simulink model "overalldesign_change_down"  (R2025b)
settings: Solver=ode4  StartTime=0.0  StopTime=1200  FixedStep=0.01  MaxStep=0.01  RelTol=1e-4
PreLoadFcn:
  | % Component data matrix: [present, weight_kg, MX_kgmm, MY_kgmm, MZ_kgmm]
  | % Rows 1-28 correspond to Excel rows 2-29
  | comp_data_mat = [
  |   1, 80,     147543.64,  -0.88,    -1622.36;    % 底盘
  |   1, 60,      73274.04, -169.26,    3359.46;    % 轮胎
  |   0,  0,             0,       0,         0;    % 前后桥(不在位)
  |   1, 45,      99639.05,  -0.495,   35241.39;    % 蒙皮
  |   1, 159,    308512.15, -0.0298,   72044.97;    % 结构骨架
  |   1, 93,     214584.20,  -1.023,   85225.94;    % 折叠机构
  |   1, 113.92, 269830.46, -1.2531,  107552.44;    % 支臂
  |   1, 45,       1371.65, -531.27,   17662.14;    % 内饰
  |   1, 13.86,   34638.76, -0.1525,   13254.18;    % 电机底座
  |   1, 30,      69816.09,   -0.33,   26989.32;    % 飞行体
  |   1, 316,    803427.47,       0,   33092.78;    % 动力电池1
  |   0, 316,            0,       0,         0;    % 动力电池2(不在位)
  |   1, 30,      75059.94,    0.21,   37410.81;    % 旋翼
  |   1, 141,    353019.16,  -1.551,  161459.10;    % 电机
  |   1, 33,      82253.26,   -0.33,   27077.13;    % 电调
  |   1, 15,             0,       0,         0;    % PDU
  |   0, 10,             0,       0,         0;    % 导线(不在位)
  |   0,  0,             0,       0,         0;    % (空)
  |   0, 90,             0,       0,         0;    % 左商载(不在位)
  |   0, 90,             0,       0,         0;    % 右商载(不在位)
  |   0, 32,             0,       0,         0;    % 飞控运控(不在位)
  | 
  | ];
  | % Lift center [X; Y; Z] in mm
  | lift_center_vec = [2506.477; 0; 1258.273];
  | % Route parameters are set directly in top-level Constant blocks:
  | %   route_mode, takeoff, hover, line_cruise, circle_cruise, land
model workspace (MAT data in the model file):
  CS_duct_lift_slew_rate = 7031250
  CS_main_rotor_slew_rate = 1567.1641791
  CS_max_acc_xy = 5
  CS_max_acc_z_down = 5
  CS_max_acc_z_up = 5
  CS_max_jerk_xy = 20
  CS_max_jerk_z_down = 20
  CS_max_jerk_z_up = 20
  CS_max_vel_xy = 20
  CS_max_vel_z_down = 20
  CS_max_vel_z_up = 20
  CS_motor_tau_duct = 0.07
  CS_motor_tau_main = 0.336
  Kd_rate_rp = 12
  Kd_rate_y = 8
  Kd_vel_xy = 1.5
  Kd_vel_z = 1
  Ki_rate_rp = 4
  Ki_rate_y = 10
  Ki_vel_xy = 0.02
  Ki_vel_z = 0.05
  Kp_att_rp = 2.5
  Kp_att_tilt = 2.5
  Kp_att_y = 1.5
  Kp_att_yaw = 1.5
  Kp_pos_xy = 0.4
  Kp_pos_z = 1
  Kp_rate_rp = 300
  Kp_rate_y = 200
  Kp_vel_xy = 1.5
  Kp_vel_z = 1.5
  P.source.audit_file = 'main_model_param_audit.xlsx'
  P.source.note = 'CG and motor positions are default snapshots here. The pipeline updates them from Excel before simulation.'
  P.model.stop_time_s = 60
  P.model.cg_calculation_commented = 'on'
  P.route.mode = 2
  P.fault.id = 0
  P.mass_kg = 1200
  P.inertia_kgm2 = [3959.6  0  0; 0  3041.4  0; 0  0  2640.2]
  P.cg_offset_m = [0.038293; -0.0063; 0.28227]
  P.environment.gravity_mps2 = 9.81
  P.environment.rho_kgpm3 = 1.225
  P.environment.g = 9.81
  P.environment.rho = 1.225
  P.battery.total_Wh = 80000
  P.battery.usable_ratio = 0.8
  P.motor.efficiency = 0.85
  P.rotor.count = 6
  P.rotor.radius_m = 1.3
  P.rotor.blade_num = 2
  P.rotor.chord_avg_m = 0.18
  P.rotor.pos_m = [2.624  -2.228  -0.465; 2.624  2.228  -0.465; 0  -2.235  0; 0  2.235  0; -2.599  -2.231  -0.464; -2.599  2.231  -0.464]
  P.rotor.spin_dir = [1; -1; -1; 1; 1; -1]
  P.rotor.kF_N_per_radps2 = 0.00141483
  P.rotor.kM_Nm_per_radps2 = 0.000167666
  P.rotor.power_coeff_W_per_radps3 = 1.74522e-05
  P.rotor.kF = 0.00141483
  P.rotor.kM = 0.000167666
  P.rotor.speed_max_radps = 1770
  P.rotor.speed_margin_radps = 1600
  P.duct.power_coeff_W_per_radps3 = 5.12708e-07
  P.duct.kF_N_per_radps2 = 4.54e-05
  P.duct.kF = 4.54e-05
  P.duct.pos_m = [3  0  0; 3  0  0]
  P.duct.force_dir = [0  -1  0; 0  1  0]
  P.mixer.T_hover_N = 11772
  P.mixer.W_hover_radps = 1177.6
  P.mixer.ref_col_norms = [2.014; 2.149; 2.4849; 2.4849]
  P.control.max_tilt_deg = 20
  P.control.max_tilt_rad = 0.349065850399
  P.review.current_6DoF_mass_kg = 1208.5
  P.review.current_Perf_Calc_mass_kg = 1208.5
  P.review.GravBlock_mass_kg = 1200
  P.review.Accel2Attitude_mass_kg = 1200
  P.review.model_workspace_cg_offset_m = [0.25; 0; 0.62]
  P.review.model_workspace_motor_pos_m = [2.592  -2.306  0; 2.592  2.306  0; 0  -2.505  0; 0  2.505  0; -2.592  -2.306  0; -2.592  2.306  0]
  T_hover = 11772
  V_descent = []
  W_hover = 1194
  W_margin = 1600
  cg_offset_m = [0.038293; -0.0063; 0.28227]
  cg_x_delta_m = 0
  climbRate_mps = 5
  cruiseSpeed_mps = 20
  descentRate_mps = 5
  duct_dir = [0  -1  0; 0  1  0]
  duct_pos_0 = [3  0  0; 3  0  0]
  fault_id = 0
  fault_mask = [0; 0; 0; 0; 0; 0; 0; 0]
  hover_x = 0
  hover_y = 0
  hover_yaw = 0
  hover_z = -120
  inertia_kgm2 = [3959.6  0  0; 0  3041.4  0; 0  0  2640.2]
  kF = 0.0013767
  kF_duct = 4.54e-05
  kM = 0.000164967
  kM_coeff = 1.72621225e-05
  kM_duct = 4.896e-06
  kM_duct_coeff = 5.12708e-07
  k_yaw_weight = 0.5
  mass_kg = 1200
  motor_coord = [2.624  -2.228  -0.465; 2.624  2.228  -0.465; 0  -2.235  0; 0  2.235  0; -2.599  -2.231  -0.464; -2.599  2.231  -0.464; 3  0  0; 3  0  0]
  motor_dir = [1; -1; -1; 1; 1; -1]
  motor_efficiency = 0.9016
  motor_pos_0 = [2.624  -2.228  -0.465; 2.624  2.228  -0.465; 0  -2.235  0; 0  2.235  0; -2.599  -2.231  -0.464; -2.599  2.231  -0.464]
  offline_opt_applyBestToModel = 1
  offline_opt_maxEvaluations = 10
  offline_opt_method = 'auto'
  offline_opt_saveBestToModel = 0
  offline_opt_updateDiagramAfterBest = 1
  perf_battery_Wh = 80000
  perf_blade_num = 2
  perf_chord_avg = 0.18
  perf_mass_kg = 1200
  perf_rho = 1.225
  perf_rotor_num = 6
  perf_rotor_radius = 1.3
  perf_usable_ratio = 0.8
  speed_max_radps = 1750
  tau_limit_rp = 2000
  tau_limit_y = 1000
  thrust_degrade = 0.7
libraries: slpidlib x6, aerolibprivatev1p5 x1, dspnetwork x1
(part 1 of 2)
settings Model: Creator=admin  LastModifiedBy=91390
settings SolverCC: ZeroCrossControl=DisableAll

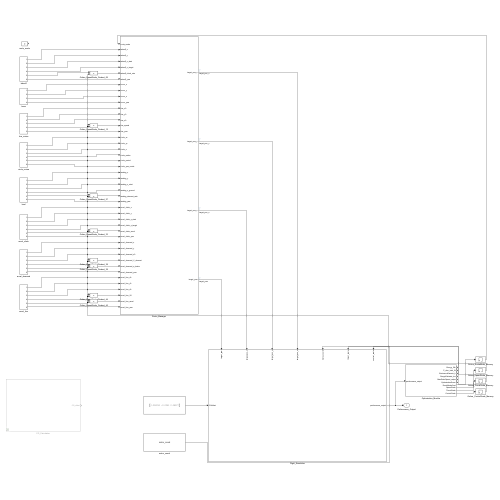
[thumbnail: Simulink's stored preview of the top-level diagram]
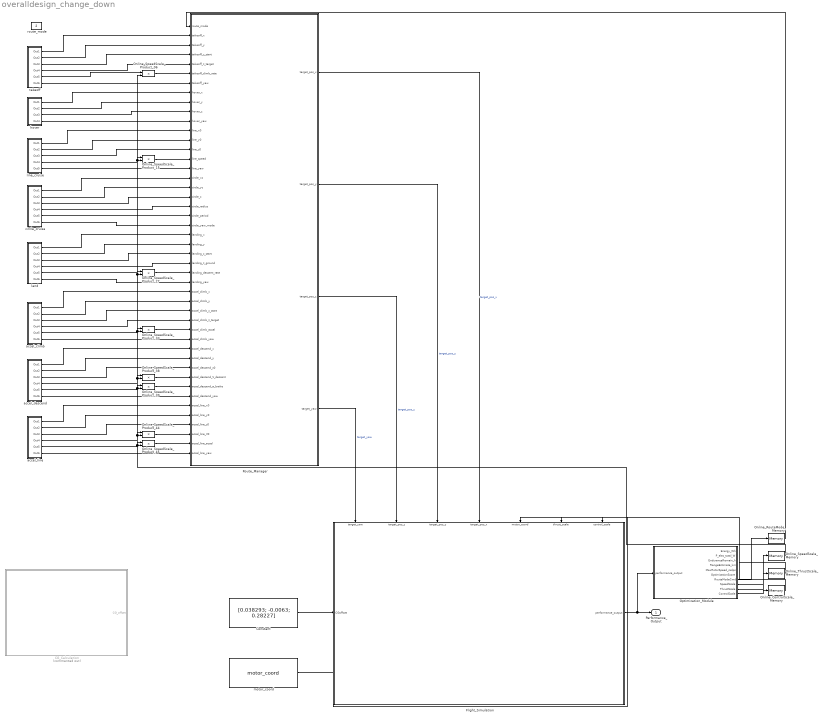
== system overalldesign_change_down ==
  CG_Calculation : Subsystem  Commented=on
  Constant : Constant  Value=[0.038293; -0.0063; 0.28227]
  Flight_Simulation : Subsystem
      settings: PortSchema="{\"entries\":[{\"content\":{\"sides\":[{\"content\":{\"connectorIds\":[\"In1\"]},\"type\":\"ConnectorPlacement.EquallySpacedRectSide\",\"uuid\":\"5deb5f2c-62ad-40f5-b613-353336255dba\"},{\"content\":{\"connectorIds\":[\"Out1\"],\"side\":\"RIGHT\"},\"type\":\"ConnectorPlacement.EquallySpacedRectSide\",\"uuid\":\"a56ec260-326c-4a45-a418-c08f727a598e\"},{\"content\":{\"connectorIds\":[\"In2\",\"In3\",\"In4\",\"In5\",\"In6\",\"In7\",\"In8\"],\"side\":\"TOP\"},\"type\":\"ConnectorPlacement.EquallySpacedRectSide\",\"uuid\":\"b9e0438d-138c-455b-afb0-6983736d76da\"}]},\"type\":\"ConnectorPlacement.EquallySpacedConnector\",\"uuid\":\"d5d418e6-8e97-46b2-8c41-4077eef2ab5a\"}],\"packageUris\":[\"http://schema.mathworks.com/mf0/Connector/R2020b\"],\"version\":\"1.0\"}"
  Online_ControlScale_Memory : Memory  InitialCondition=1
  Online_RouteMode_Memory : Memory  InitialCondition=1
  Online_SpeedScale_Memory : Memory  InitialCondition=1
  Online_SpeedScale_Product_06 : Product
  Online_SpeedScale_Product_{15,27,33,38..39,44..45} (7 alike) : Product
  Online_ThrustScale_Memory : Memory  InitialCondition=1
  Optimization_Module : Subsystem
  Route_Manager : Subsystem
  accel_climb : Subsystem
  accel_descend : Subsystem
  accel_line : Subsystem
  circle_cruise : Subsystem
  hover : Subsystem
  land : Subsystem
  line_cruise : Subsystem
  motor_coord : Constant  Value=motor_coord
  route_mode : Constant  Value=2
  takeoff : Subsystem
  Performance_Output : Outport
  wires:
  line_cruise/5(Out5) -> Route_Manager/16(line_yaw)
  takeoff/4(Out4) -> Route_Manager/5(takeoff_z_target)
  takeoff/1(Out1) -> Route_Manager/2(takeoff_x)
  circle_cruise/2(Out2) -> Route_Manager/18(circle_yc)
  takeoff/6(Out6) -> Route_Manager/7(takeoff_yaw)
  takeoff/2(Out2) -> Route_Manager/3(takeoff_y)
  accel_line/6(Out6) -> Route_Manager/46(accel_line_yaw)
  takeoff/3(Out3) -> Route_Manager/4(takeoff_z_start)
  hover/1(Out1) -> Route_Manager/8(hover_x)
  hover/2(Out2) -> Route_Manager/9(hover_y)
  hover/3(Out3) -> Route_Manager/10(hover_z)
  accel_descend/6(Out6) -> Route_Manager/40(accel_descend_yaw)
  hover/4(Out4) -> Route_Manager/11(hover_yaw)
  accel_descend/1(Out1) -> Route_Manager/35(accel_descend_x)
  accel_climb/4(Out4) -> Route_Manager/32(accel_climb_z_target)
  line_cruise/1(Out1) -> Route_Manager/12(line_x0)
  line_cruise/2(Out2) -> Route_Manager/13(line_y0)
  circle_cruise/6(Out6) -> Route_Manager/22(circle_yaw_mode)
  line_cruise/3(Out3) -> Route_Manager/14(line_z0)
  circle_cruise/1(Out1) -> Route_Manager/17(circle_xc)
  circle_cruise/3(Out3) -> Route_Manager/19(circle_z)
  circle_cruise/4(Out4) -> Route_Manager/20(circle_radius)
  accel_line/3(Out3) -> Route_Manager/43(accel_line_z0)
  circle_cruise/5(Out5) -> Route_Manager/21(circle_period)
  land/1(Out1) -> Route_Manager/23(landing_x)
  land/2(Out2) -> Route_Manager/24(landing_y)
  land/3(Out3) -> Route_Manager/25(landing_z_start)
  land/4(Out4) -> Route_Manager/26(landing_z_ground)
  accel_descend/3(Out3) -> Route_Manager/37(accel_descend_z0)
  land/6(Out6) -> Route_Manager/28(landing_yaw)
  accel_climb/1(Out1) -> Route_Manager/29(accel_climb_x)
  accel_climb/2(Out2) -> Route_Manager/30(accel_climb_y)
  accel_climb/3(Out3) -> Route_Manager/31(accel_climb_z_start)
  accel_climb/6(Out6) -> Route_Manager/34(accel_climb_yaw)
  accel_descend/2(Out2) -> Route_Manager/36(accel_descend_y)
  accel_line/1(Out1) -> Route_Manager/41(accel_line_x0)
  accel_line/2(Out2) -> Route_Manager/42(accel_line_y0)
  Constant/1 -> Flight_Simulation/1(CGoffset)
  Route_Manager/4(target_yaw) -> Flight_Simulation/2(target_yaw)  "target_yaw"
  Route_Manager/3(target_pos_z) -> Flight_Simulation/3(target_pos_z)  "target_pos_z"
  Route_Manager/2(target_pos_y) -> Flight_Simulation/4(target_pos_y)  "target_pos_y"
  Route_Manager/1(target_pos_x) -> Flight_Simulation/5(target_pos_x)  "target_pos_x"
  motor_coord/1 -> Flight_Simulation/6(motor_coord)
  Flight_Simulation/1(performance_output) -> Performance_Output/1, Optimization_Module/1(performance_output)
  Optimization_Module/7(RouteModeCmd) -> Online_RouteMode_Memory/1
  Optimization_Module/8(SpeedScale) -> Online_SpeedScale_Memory/1
  Optimization_Module/9(ThrustScale) -> Online_ThrustScale_Memory/1
  Optimization_Module/10(ControlScale) -> Online_ControlScale_Memory/1
  Online_RouteMode_Memory/1 -> Route_Manager/1(route_mode)
  Online_ThrustScale_Memory/1 -> Flight_Simulation/7(thrust_scale)
  Online_ControlScale_Memory/1 -> Flight_Simulation/8(control_scale)
  takeoff/5(Out5) -> Online_SpeedScale_Product_06/1
  Online_SpeedScale_Memory/1 -> Online_SpeedScale_Product_06/2, Online_SpeedScale_Product_15/2, Online_SpeedScale_Product_27/2, Online_SpeedScale_Product_33/2, Online_SpeedScale_Product_38/2, Online_SpeedScale_Product_39/2, Online_SpeedScale_Product_44/2, Online_SpeedScale_Product_45/2
  Online_SpeedScale_Product_06/1 -> Route_Manager/6(takeoff_climb_rate)
  line_cruise/4(Out4) -> Online_SpeedScale_Product_15/1
  Online_SpeedScale_Product_15/1 -> Route_Manager/15(line_speed)
  land/5(Out5) -> Online_SpeedScale_Product_27/1
  Online_SpeedScale_Product_27/1 -> Route_Manager/27(landing_descent_rate)
  accel_climb/5(Out5) -> Online_SpeedScale_Product_33/1
  Online_SpeedScale_Product_33/1 -> Route_Manager/33(accel_climb_accel)
  accel_descend/4(Out4) -> Online_SpeedScale_Product_38/1
  Online_SpeedScale_Product_38/1 -> Route_Manager/38(accel_descend_V_descent)
  accel_descend/5(Out5) -> Online_SpeedScale_Product_39/1
  Online_SpeedScale_Product_39/1 -> Route_Manager/39(accel_descend_a_brake)
  accel_line/4(Out4) -> Online_SpeedScale_Product_44/1
  Online_SpeedScale_Product_44/1 -> Route_Manager/44(accel_line_V0)
  accel_line/5(Out5) -> Online_SpeedScale_Product_45/1
  Online_SpeedScale_Product_45/1 -> Route_Manager/45(accel_line_accel)

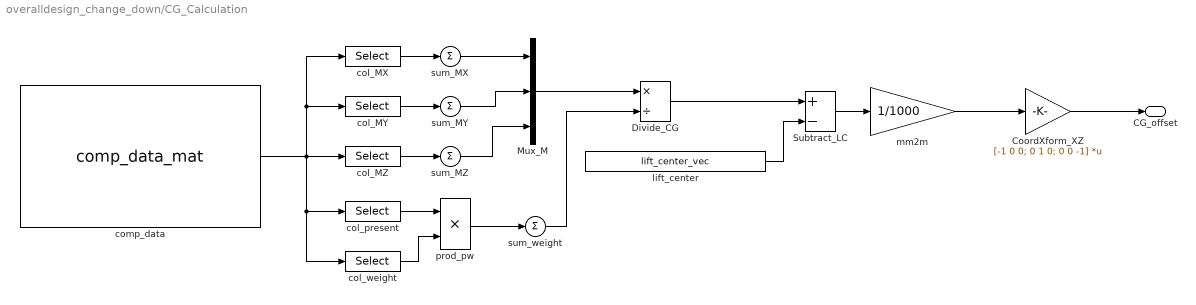
== system overalldesign_change_down/CG_Calculation ==
  CoordXform_XZ : Gain  Gain=[-1 0 0; 0 1 0; 0 0 -1]  Multiplication=Matrix(K*u)
  Divide_CG : Product  Inputs=*/
  Mux_M : Mux  Inputs=3
  Subtract_LC : Sum  Inputs=+-
  col_MX : Selector  NumberOfDimensions=2  InputPortWidth=3  IndexOptions=Select all,Index vector (dialog)  Indices=Select all,[3]  OutputSizes=1
  col_MY : Selector  NumberOfDimensions=2  InputPortWidth=3  IndexOptions=Select all,Index vector (dialog)  Indices=Select all,[4]  OutputSizes=1
  col_MZ : Selector  NumberOfDimensions=2  InputPortWidth=3  IndexOptions=Select all,Index vector (dialog)  Indices=Select all,[5]  OutputSizes=1
  col_present : Selector  NumberOfDimensions=2  InputPortWidth=3  IndexOptions=Select all,Index vector (dialog)  Indices=Select all,[1]  OutputSizes=1
  col_weight : Selector  NumberOfDimensions=2  InputPortWidth=3  IndexOptions=Select all,Index vector (dialog)  Indices=Select all,[2]  OutputSizes=1
  comp_data : Constant  Value=comp_data_mat
  lift_center : Constant  Value=lift_center_vec
  mm2m : Gain  Gain=1/1000
  prod_pw : Product
  sum_MX : Sum  Inputs=+
  sum_MY : Sum  Inputs=+
  sum_MZ : Sum  Inputs=+
  sum_weight : Sum  Inputs=+
  CG_offset : Outport
  wires:
  comp_data/1 -> col_MX/1, col_MY/1, col_weight/1, col_present/1, col_MZ/1
  col_weight/1 -> prod_pw/2
  Subtract_LC/1 -> mm2m/1
  col_MX/1 -> sum_MX/1
  col_MY/1 -> sum_MY/1
  col_present/1 -> prod_pw/1
  col_MZ/1 -> sum_MZ/1
  sum_MY/1 -> Mux_M/2
  sum_MX/1 -> Mux_M/1
  sum_MZ/1 -> Mux_M/3
  prod_pw/1 -> sum_weight/1
  Mux_M/1 -> Divide_CG/1
  sum_weight/1 -> Divide_CG/2
  Divide_CG/1 -> Subtract_LC/1
  lift_center/1 -> Subtract_LC/2
  mm2m/1 -> CoordXform_XZ/1
  CoordXform_XZ/1 -> CG_offset/1

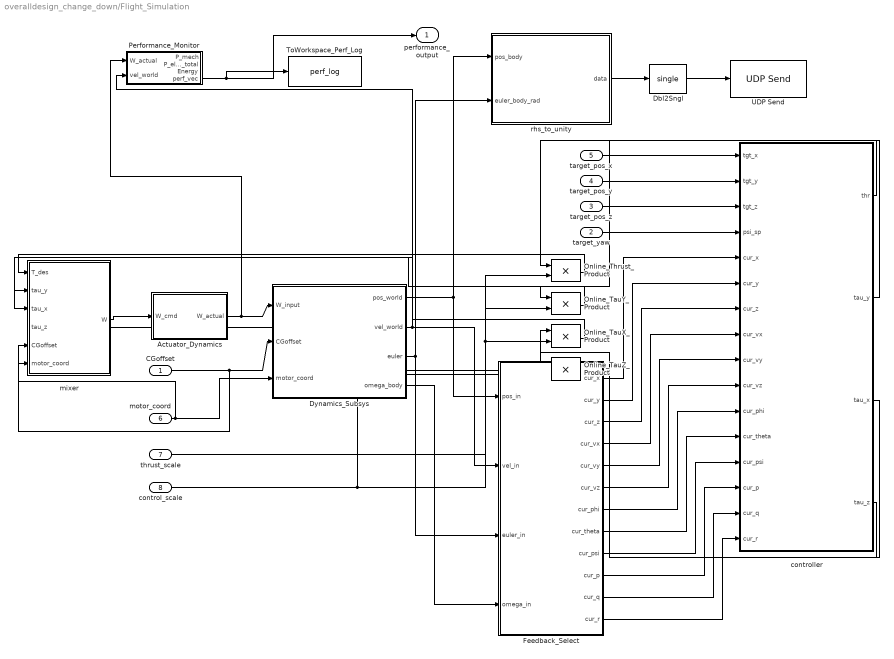
== system overalldesign_change_down/Flight_Simulation ==
  CGoffset : Inport  PortDimensions=3
  target_yaw : Inport  Port=2
  target_pos_z : Inport  Port=3
  target_pos_y : Inport  Port=4
  target_pos_x : Inport  Port=5
  motor_coord : Inport  Port=6
  thrust_scale : Inport  Port=7
  control_scale : Inport  Port=8
  Actuator_Dynamics : Subsystem
  Dbl2Sngl : DataTypeConversion  OutDataTypeStr=single  SaturateOnIntegerOverflow=off  RndMeth=Floor
  Dynamics_Subsys : Subsystem
  Feedback_Select : Subsystem
  Online_TauX_Product : Product
  Online_TauY_Product : Product
  Online_TauZ_Product : Product
  Online_Thrust_Product : Product
  Performance_Monitor : Subsystem
  ToWorkspace_Perf_Log : ToWorkspace  VariableName=perf_log  SaveFormat=Timeseries  SampleTime=-1
  UDP Send : dspnetwork/UDP Send  remoteURL='127.0.0.1'  remotePort=23334  localURL='0.0.0.0'  localPortSource=Automatically determine  localPort=-1  sendBufferSize=512  sampletime=-1  blockPlatform=[]  separateLengthPort=0
  controller : Subsystem
  mixer : Subsystem
  rhs_to_unity : MATLAB Function  TreatAsAtomicUnit=on
  performance_output : Outport
  wires:
  rhs_to_unity/1(data) -> Dbl2Sngl/1
  Feedback_Select/1(cur_x) -> controller/5(cur_x)
  Dynamics_Subsys/1(pos_world) -> rhs_to_unity/1(pos_body), Feedback_Select/1(pos_in)
  Dynamics_Subsys/3(euler) -> rhs_to_unity/2(euler_body_rad), Feedback_Select/3(euler_in)
  Feedback_Select/9(cur_psi) -> controller/13(cur_psi)
  Feedback_Select/10(cur_p) -> controller/14(cur_p)
  Feedback_Select/7(cur_phi) -> controller/11(cur_phi)
  Dbl2Sngl/1 -> UDP Send/1
  Dynamics_Subsys/2(vel_world) -> Feedback_Select/2(vel_in), Performance_Monitor/2(vel_world)
  mixer/1(W) -> Actuator_Dynamics/1(W_cmd)
  Feedback_Select/2(cur_y) -> controller/6(cur_y)
  Feedback_Select/11(cur_q) -> controller/15(cur_q)
  Feedback_Select/6(cur_vz) -> controller/10(cur_vz)
  Feedback_Select/3(cur_z) -> controller/7(cur_z)
  Dynamics_Subsys/4(omega_body) -> Feedback_Select/4(omega_in)
  Feedback_Select/5(cur_vy) -> controller/9(cur_vy)
  Feedback_Select/12(cur_r) -> controller/16(cur_r)
  Feedback_Select/4(cur_vx) -> controller/8(cur_vx)
  Feedback_Select/8(cur_theta) -> controller/12(cur_theta)
  target_pos_x/1 -> controller/1(tgt_x)
  target_pos_y/1 -> controller/2(tgt_y)
  target_pos_z/1 -> controller/3(tgt_z)
  target_yaw/1 -> controller/4(psi_sp)
  CGoffset/1 -> Dynamics_Subsys/2(CGoffset), mixer/5(CGoffset)
  Actuator_Dynamics/1(W_actual) -> Dynamics_Subsys/1(W_input), Performance_Monitor/1(W_actual)
  Performance_Monitor/4(perf_vec) -> ToWorkspace_Perf_Log/1, performance_output/1
  motor_coord/1 -> mixer/6(motor_coord), Dynamics_Subsys/3(motor_coord)
  controller/1(thr) -> Online_Thrust_Product/1
  thrust_scale/1 -> Online_Thrust_Product/2
  Online_Thrust_Product/1 -> mixer/1(T_des)
  controller/2(tau_y) -> Online_TauY_Product/1
  control_scale/1 -> Online_TauY_Product/2, Online_TauX_Product/2, Online_TauZ_Product/2
  Online_TauY_Product/1 -> mixer/2(tau_y)
  controller/3(tau_x) -> Online_TauX_Product/1
  Online_TauX_Product/1 -> mixer/3(tau_x)
  controller/4(tau_z) -> Online_TauZ_Product/1
  Online_TauZ_Product/1 -> mixer/4(tau_z)

== system overalldesign_change_down/Optimization_Module ==
  performance_output : Inport
  MetricsMux : Mux  Inputs=10
  ToWorkspace_Optimization_Log : ToWorkspace  VariableName=optimization_metrics_log  SaveFormat=Timeseries  SampleTime=-1
  extract_metrics : MATLAB Function  TreatAsAtomicUnit=on
  Energy_Wh : Outport
  P_elec_total_W : Outport  Port=2
  EnduranceRemain_h : Outport  Port=3
  RangeEstimate_km : Outport  Port=4
  MaxRotorSpeed_radps : Outport  Port=5
  OptimizationScore : Outport  Port=6
  RouteModeCmd : Outport  Port=7
  SpeedScale : Outport  Port=8
  ThrustScale : Outport  Port=9
  ControlScale : Outport  Port=10
  wires:
  performance_output/1 -> extract_metrics/1(performance_output)
  extract_metrics/1(Energy_Wh) -> Energy_Wh/1, MetricsMux/1
  extract_metrics/2(P_elec_total_W) -> P_elec_total_W/1, MetricsMux/2
  extract_metrics/3(EnduranceRemain_h) -> EnduranceRemain_h/1, MetricsMux/3
  extract_metrics/4(RangeEstimate_km) -> RangeEstimate_km/1, MetricsMux/4
  extract_metrics/5(MaxRotorSpeed_radps) -> MaxRotorSpeed_radps/1, MetricsMux/5
  extract_metrics/6(OptimizationScore) -> OptimizationScore/1, MetricsMux/6
  MetricsMux/1 -> ToWorkspace_Optimization_Log/1
  extract_metrics/7(RouteModeCmd) -> RouteModeCmd/1, MetricsMux/7
  extract_metrics/8(SpeedScale) -> SpeedScale/1, MetricsMux/8
  extract_metrics/9(ThrustScale) -> ThrustScale/1, MetricsMux/9
  extract_metrics/10(ControlScale) -> ControlScale/1, MetricsMux/10

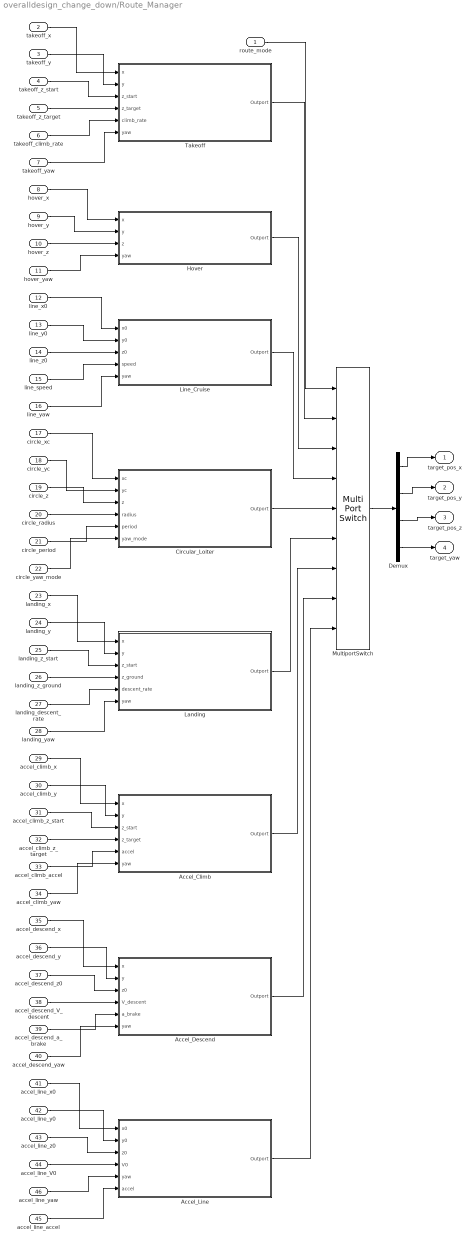
== system overalldesign_change_down/Route_Manager ==
  route_mode : Inport
  takeoff_x : Inport  Port=2
  takeoff_y : Inport  Port=3
  takeoff_z_start : Inport  Port=4
  takeoff_z_target : Inport  Port=5
  takeoff_climb_rate : Inport  Port=6
  takeoff_yaw : Inport  Port=7
  hover_x : Inport  Port=8
  hover_y : Inport  Port=9
  hover_z : Inport  Port=10
  hover_yaw : Inport  Port=11
  line_x0 : Inport  Port=12
  line_y0 : Inport  Port=13
  line_z0 : Inport  Port=14
  line_speed : Inport  Port=15
  line_yaw : Inport  Port=16
  circle_xc : Inport  Port=17
  circle_yc : Inport  Port=18
  circle_z : Inport  Port=19
  circle_radius : Inport  Port=20
  circle_period : Inport  Port=21
  circle_yaw_mode : Inport  Port=22
  landing_x : Inport  Port=23
  landing_y : Inport  Port=24
  landing_z_start : Inport  Port=25
  landing_z_ground : Inport  Port=26
  landing_descent_rate : Inport  Port=27
  landing_yaw : Inport  Port=28
  accel_climb_x : Inport  Port=29
  accel_climb_y : Inport  Port=30
  accel_climb_z_start : Inport  Port=31
  accel_climb_z_target : Inport  Port=32
  accel_climb_accel : Inport  Port=33
  accel_climb_yaw : Inport  Port=34
  accel_descend_x : Inport  Port=35
  accel_descend_y : Inport  Port=36
  accel_descend_z0 : Inport  Port=37
  accel_descend_V_descent : Inport  Port=38
  accel_descend_a_brake : Inport  Port=39
  accel_descend_yaw : Inport  Port=40
  accel_line_x0 : Inport  Port=41
  accel_line_y0 : Inport  Port=42
  accel_line_z0 : Inport  Port=43
  accel_line_V0 : Inport  Port=44
  accel_line_accel : Inport  Port=45
  accel_line_yaw : Inport  Port=46
  Accel_Climb : Subsystem
  Accel_Descend : Subsystem
  Accel_Line : Subsystem
  Circular_Loiter : Subsystem
  Demux : Demux
  Hover : Subsystem
  Landing : Subsystem
  Line_Cruise : Subsystem
  MultiportSwitch : MultiPortSwitch  Inputs=8  DataPortIndices={1,2,3,4,5,6,7,8}  SaturateOnIntegerOverflow=off  InputSameDT=off
  Takeoff : Subsystem
  target_pos_x : Outport
  target_pos_y : Outport  Port=2
  target_pos_z : Outport  Port=3
  target_yaw : Outport  Port=4
  wires:
  takeoff_climb_rate/1 -> Takeoff/5(climb_rate)
  Line_Cruise/1(Outport) -> MultiportSwitch/4
  accel_line_y0/1 -> Accel_Line/2(y0)
  accel_climb_yaw/1 -> Accel_Climb/6(yaw)
  takeoff_x/1 -> Takeoff/1(x)
  takeoff_yaw/1 -> Takeoff/6(yaw)
  accel_line_z0/1 -> Accel_Line/3(z0)
  accel_descend_x/1 -> Accel_Descend/1(x)
  takeoff_y/1 -> Takeoff/2(y)
  accel_climb_z_target/1 -> Accel_Climb/4(z_target)
  hover_x/1 -> Hover/1(x)
  accel_descend_y/1 -> Accel_Descend/2(y)
  line_yaw/1 -> Line_Cruise/5(yaw)
  takeoff_z_start/1 -> Takeoff/3(z_start)
  hover_y/1 -> Hover/2(y)
  accel_line_accel/1 -> Accel_Line/6(accel)
  takeoff_z_target/1 -> Takeoff/4(z_target)
  circle_yaw_mode/1 -> Circular_Loiter/6(yaw_mode)
  hover_z/1 -> Hover/3(z)
  hover_yaw/1 -> Hover/4(yaw)
  line_x0/1 -> Line_Cruise/1(x0)
  accel_descend_z0/1 -> Accel_Descend/3(z0)
  line_y0/1 -> Line_Cruise/2(y0)
  accel_line_yaw/1 -> Accel_Line/5(yaw)
  line_z0/1 -> Line_Cruise/3(z0)
  landing_x/1 -> Landing/1(x)
  line_speed/1 -> Line_Cruise/4(speed)
  Landing/1(Outport) -> MultiportSwitch/6
  circle_xc/1 -> Circular_Loiter/1(xc)
  Accel_Climb/1(Outport) -> MultiportSwitch/7
  circle_yc/1 -> Circular_Loiter/2(yc)
  accel_climb_z_start/1 -> Accel_Climb/3(z_start)
  circle_z/1 -> Circular_Loiter/3(z)
  circle_radius/1 -> Circular_Loiter/4(radius)
  MultiportSwitch/1 -> Demux/1
  route_mode/1 -> MultiportSwitch/1
  accel_line_x0/1 -> Accel_Line/1(x0)
  circle_period/1 -> Circular_Loiter/5(period)
  accel_line_V0/1 -> Accel_Line/4(V0)
  landing_y/1 -> Landing/2(y)
  landing_z_start/1 -> Landing/3(z_start)
  landing_z_ground/1 -> Landing/4(z_ground)
  landing_descent_rate/1 -> Landing/5(descent_rate)
  accel_descend_yaw/1 -> Accel_Descend/6(yaw)
  landing_yaw/1 -> Landing/6(yaw)
  accel_climb_x/1 -> Accel_Climb/1(x)
  accel_descend_V_descent/1 -> Accel_Descend/4(V_descent)
  accel_climb_y/1 -> Accel_Climb/2(y)
  accel_climb_accel/1 -> Accel_Climb/5(accel)
  accel_descend_a_brake/1 -> Accel_Descend/5(a_brake)
  Takeoff/1(Outport) -> MultiportSwitch/2
  Hover/1(Outport) -> MultiportSwitch/3
  Circular_Loiter/1(Outport) -> MultiportSwitch/5
  Accel_Descend/1(Outport) -> MultiportSwitch/8
  Accel_Line/1(Outport) -> MultiportSwitch/9
  Demux/1 -> target_pos_x/1
  Demux/4 -> target_yaw/1
  Demux/3 -> target_pos_z/1
  Demux/2 -> target_pos_y/1

== system overalldesign_change_down/accel_climb ==
  accel_climb_accel : Constant  Value=0.981
  accel_climb_x : Constant  Value=0
  accel_climb_y : Constant  Value=0
  accel_climb_yaw : Constant  Value=0
  accel_climb_z_start : Constant  Value=-10
  accel_climb_z_target : Constant  Value=-1000
  Out1 : Outport
  Out2 : Outport  Port=2
  Out3 : Outport  Port=3
  Out4 : Outport  Port=4
  Out5 : Outport  Port=5
  Out6 : Outport  Port=6
  wires:
  accel_climb_x/1 -> Out1/1
  accel_climb_y/1 -> Out2/1
  accel_climb_z_start/1 -> Out3/1
  accel_climb_z_target/1 -> Out4/1
  accel_climb_accel/1 -> Out5/1
  accel_climb_yaw/1 -> Out6/1

== system overalldesign_change_down/accel_descend ==
  V_descent : Constant  Value=10
  a_brake : Constant  Value=2.4525
  x0 : Constant  Value=0
  y0 : Constant  Value=0
  yaw : Constant  Value=0
  z0 : Constant  Value=-10
  Out1 : Outport
  Out2 : Outport  Port=2
  Out3 : Outport  Port=3
  Out4 : Outport  Port=4
  Out5 : Outport  Port=5
  Out6 : Outport  Port=6
  wires:
  x0/1 -> Out1/1
  y0/1 -> Out2/1
  z0/1 -> Out3/1
  V_descent/1 -> Out4/1
  a_brake/1 -> Out5/1
  yaw/1 -> Out6/1

== system overalldesign_change_down/accel_line ==
  accel_line_V0 : Constant  Value=0
  accel_line_accel : Constant  Value=2.4525
  accel_line_x0 : Constant  Value=0
  accel_line_y0 : Constant  Value=0
  accel_line_yaw : Constant  Value=0
  accel_line_z0 : Constant  Value=-10
  Out1 : Outport
  Out2 : Outport  Port=2
  Out3 : Outport  Port=3
  Out4 : Outport  Port=4
  Out5 : Outport  Port=5
  Out6 : Outport  Port=6
  wires:
  accel_line_x0/1 -> Out1/1
  accel_line_y0/1 -> Out2/1
  accel_line_z0/1 -> Out3/1
  accel_line_V0/1 -> Out4/1
  accel_line_accel/1 -> Out5/1
  accel_line_yaw/1 -> Out6/1

== system overalldesign_change_down/circle_cruise ==
  circle_altZ : Constant  Value=-10
  circle_ctrX : Constant  Value=-30
  circle_ctrY : Constant  Value=0
  circle_period : Constant  Value=60
  circle_radius : Constant  Value=20
  circle_yawMode : Constant
  Out1 : Outport
  Out2 : Outport  Port=2
  Out3 : Outport  Port=3
  Out4 : Outport  Port=4
  Out5 : Outport  Port=5
  Out6 : Outport  Port=6
  wires:
  circle_radius/1 -> Out4/1
  circle_ctrY/1 -> Out2/1
  circle_yawMode/1 -> Out6/1
  circle_ctrX/1 -> Out1/1
  circle_altZ/1 -> Out3/1
  circle_period/1 -> Out5/1

== system overalldesign_change_down/hover ==
  hover_X : Constant  Value=0
  hover_Y : Constant  Value=0
  hover_Yaw : Constant  Value=0.785
  hover_Z : Constant  Value=-10
  Out1 : Outport
  Out2 : Outport  Port=2
  Out3 : Outport  Port=3
  Out4 : Outport  Port=4
  wires:
  hover_Z/1 -> Out3/1
  hover_Yaw/1 -> Out4/1
  hover_X/1 -> Out1/1
  hover_Y/1 -> Out2/1

== system overalldesign_change_down/land ==
  landing_Vdesc : Constant  Value=descentRate_mps
  landing_X : Constant  Value=21440
  landing_Y : Constant  Value=0
  landing_Yaw : Constant  Value=0
  landing_Zgnd : Constant  Value=0
  landing_Zstart : Constant  Value=-300
  Out1 : Outport
  Out2 : Outport  Port=2
  Out3 : Outport  Port=3
  Out4 : Outport  Port=4
  Out5 : Outport  Port=5
  Out6 : Outport  Port=6
  wires:
  landing_X/1 -> Out1/1
  landing_Vdesc/1 -> Out5/1
  landing_Zstart/1 -> Out3/1
  landing_Y/1 -> Out2/1
  landing_Yaw/1 -> Out6/1
  landing_Zgnd/1 -> Out4/1

== system overalldesign_change_down/line_cruise ==
  line_Vcruise : Constant  Value=cruiseSpeed_mps
  line_altZ : Constant  Value=-300
  line_heading : Constant  Value=0
  line_startX : Constant  Value=0
  line_startY : Constant  Value=0
  Out1 : Outport
  Out2 : Outport  Port=2
  Out3 : Outport  Port=3
  Out4 : Outport  Port=4
  Out5 : Outport  Port=5
  wires:
  line_altZ/1 -> Out3/1
  line_heading/1 -> Out5/1
  line_startY/1 -> Out2/1
  line_startX/1 -> Out1/1
  line_Vcruise/1 -> Out4/1

== system overalldesign_change_down/takeoff ==
  takeoff_Vclimb : Constant  Value=climbRate_mps
  takeoff_X : Constant  Value=0
  takeoff_Y : Constant  Value=0
  takeoff_Yaw : Constant  Value=0
  takeoff_Zstart : Constant  Value=0
  takeoff_Ztgt : Constant  Value=-300
  Out1 : Outport
  Out2 : Outport  Port=2
  Out3 : Outport  Port=3
  Out4 : Outport  Port=4
  Out5 : Outport  Port=5
  Out6 : Outport  Port=6
  wires:
  takeoff_Yaw/1 -> Out6/1
  takeoff_Vclimb/1 -> Out5/1
  takeoff_Y/1 -> Out2/1
  takeoff_Ztgt/1 -> Out4/1
  takeoff_Zstart/1 -> Out3/1
  takeoff_X/1 -> Out1/1

== system overalldesign_change_down/Flight_Simulation/Actuator_Dynamics ==
  note: Phase 3 actuator dynamics:
      | Main 1-6: State-Space = 1/(CS_motor_tau_main*s+1)
      | Duct 7-8: State-Space = 1/(CS_motor_tau_duct*s+1)
      | Slew limits: CS_main_rotor_slew_rate, CS_duct_lift_slew_rate
  W_cmd : Inport
  Combine_W : Mux  Inputs=2
  Duct_LiftEq_to_W : Math  Operator=sqrt
  Duct_Lift_Linear_Ramp : RateLimiter  RisingSlewLimit=CS_duct_lift_slew_rate  FallingSlewLimit=-CS_duct_lift_slew_rate  SampleTimeMode=inherited  InitialCondition=2442969
  Duct_Rotor_FirstOrder_Lag : StateSpace  A=-(1/CS_motor_tau_duct)*eye(2)  B=(1/CS_motor_tau_duct)*eye(2)  C=eye(2)  D=zeros(2)  InitialCondition=zeros(2,1)
  Duct_W_to_LiftEq : Math  Operator=square
  Main_Rotor_FirstOrder_Lag : StateSpace  A=-(1/CS_motor_tau_main)*eye(6)  B=(1/CS_motor_tau_main)*eye(6)  C=eye(6)  D=zeros(6)  InitialCondition=zeros(6,1)
  Main_Rotor_Speed_Ramp : RateLimiter  RisingSlewLimit=CS_main_rotor_slew_rate  FallingSlewLimit=-CS_main_rotor_slew_rate  SampleTimeMode=inherited  InitialCondition=W_hover
  Select_Duct_W_7_8 : Selector  InputPortWidth=8  IndexOptions=Index vector (dialog)  Indices=7:8  OutputSizes=1
  Select_Main_W_1_6 : Selector  InputPortWidth=8  IndexOptions=Index vector (dialog)  Indices=1:6  OutputSizes=1
  W_actual : Outport
  wires:
  W_cmd/1 -> Select_Main_W_1_6/1, Select_Duct_W_7_8/1
  Select_Main_W_1_6/1 -> Main_Rotor_Speed_Ramp/1
  Select_Duct_W_7_8/1 -> Duct_W_to_LiftEq/1
  Duct_W_to_LiftEq/1 -> Duct_Lift_Linear_Ramp/1
  Duct_Lift_Linear_Ramp/1 -> Duct_LiftEq_to_W/1
  Combine_W/1 -> W_actual/1  "W_actual"
  Main_Rotor_Speed_Ramp/1 -> Main_Rotor_FirstOrder_Lag/1
  Main_Rotor_FirstOrder_Lag/1 -> Combine_W/1
  Duct_LiftEq_to_W/1 -> Duct_Rotor_FirstOrder_Lag/1
  Duct_Rotor_FirstOrder_Lag/1 -> Combine_W/2

== system overalldesign_change_down/Flight_Simulation/Dynamics_Subsys ==
  W_input : Inport  PortDimensions=8
  CGoffset : Inport  Port=2  PortDimensions=3
  motor_coord : Inport  Port=3
  6DoF : aerolibprivatev1p5/6DoF (Euler Angles)  xme_0=[0; 0; 0]  Vm_0=[0; 0; 0]  eul_0=[0; 0; 0]  pm_0=[0; 0; 0]  Mass=1200  Inertia=[3959.6, 0, 0; 0, 3041.4, 0; 0, 0, 2640.2]
  Aero_Model : Subsystem
  ForceSum : Sum  Inputs=+++
  GravBlock : MATLAB Function  TreatAsAtomicUnit=on
  MomentSum : Sum  Inputs=|++
  Reshape_F : Reshape
  Reshape_M : Reshape
  Term_Ab : Terminator
  Term_DCM : Terminator
  motor_model : MATLAB Function  TreatAsAtomicUnit=on
  pos_world : Outport  PortDimensions=3
  vel_world : Outport  Port=2  PortDimensions=3
  euler : Outport  Port=3  PortDimensions=3
  omega_body : Outport  Port=4  PortDimensions=3
  wires:
  W_input/1 -> motor_model/1(W)
  motor_model/1(F_body) -> Reshape_F/1
  motor_model/2(M_body) -> Reshape_M/1
  ForceSum/1 -> 6DoF/1
  Reshape_F/1 -> ForceSum/1
  GravBlock/1(F_grav) -> ForceSum/3
  6DoF/2 -> pos_world/1
  6DoF/3 -> GravBlock/1(euler), Aero_Model/2(euler), euler/1
  6DoF/4 -> Term_DCM/1
  6DoF/6 -> omega_body/1
  6DoF/7 -> Term_Ab/1
  CGoffset/1 -> motor_model/2(CGoffset)
  Aero_Model/1(F_aero) -> ForceSum/2
  6DoF/1 -> vel_world/1
  6DoF/5 -> Aero_Model/1(V_body)
  motor_coord/1 -> motor_model/3(motor_coord)
  Reshape_M/1 -> MomentSum/2
  Aero_Model/2(M_aero) -> MomentSum/1
  MomentSum/1 -> 6DoF/2

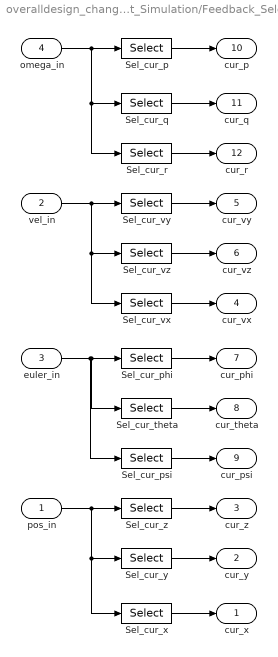
== system overalldesign_change_down/Flight_Simulation/Feedback_Select ==
  pos_in : Inport  PortDimensions=3
  vel_in : Inport  Port=2  PortDimensions=3
  euler_in : Inport  Port=3  PortDimensions=3
  omega_in : Inport  Port=4  PortDimensions=3
  Sel_cur_p : Selector  InputPortWidth=3  IndexOptions=Index vector (dialog)  Indices=1  OutputSizes=1
  Sel_cur_phi : Selector  InputPortWidth=3  IndexOptions=Index vector (dialog)  Indices=1  OutputSizes=1
  Sel_cur_psi : Selector  InputPortWidth=3  IndexOptions=Index vector (dialog)  Indices=3  OutputSizes=1
  Sel_cur_q : Selector  InputPortWidth=3  IndexOptions=Index vector (dialog)  Indices=2  OutputSizes=1
  Sel_cur_r : Selector  InputPortWidth=3  IndexOptions=Index vector (dialog)  Indices=3  OutputSizes=1
  Sel_cur_theta : Selector  InputPortWidth=3  IndexOptions=Index vector (dialog)  Indices=2  OutputSizes=1
  Sel_cur_vx : Selector  InputPortWidth=3  IndexOptions=Index vector (dialog)  Indices=1  OutputSizes=1
  Sel_cur_vy : Selector  InputPortWidth=3  IndexOptions=Index vector (dialog)  Indices=2  OutputSizes=1
  Sel_cur_vz : Selector  InputPortWidth=3  IndexOptions=Index vector (dialog)  Indices=3  OutputSizes=1
  Sel_cur_x : Selector  InputPortWidth=3  IndexOptions=Index vector (dialog)  Indices=1  OutputSizes=1
  Sel_cur_y : Selector  InputPortWidth=3  IndexOptions=Index vector (dialog)  Indices=2  OutputSizes=1
  Sel_cur_z : Selector  InputPortWidth=3  IndexOptions=Index vector (dialog)  Indices=3  OutputSizes=1
  cur_x : Outport
  cur_y : Outport  Port=2
  cur_z : Outport  Port=3
  cur_vx : Outport  Port=4
  cur_vy : Outport  Port=5
  cur_vz : Outport  Port=6
  cur_phi : Outport  Port=7
  cur_theta : Outport  Port=8
  cur_psi : Outport  Port=9
  cur_p : Outport  Port=10
  cur_q : Outport  Port=11
  cur_r : Outport  Port=12
  wires:
  Sel_cur_psi/1 -> cur_psi/1
  omega_in/1 -> Sel_cur_q/1, Sel_cur_r/1, Sel_cur_p/1
  euler_in/1 -> Sel_cur_phi/1, Sel_cur_theta/1, Sel_cur_psi/1
  Sel_cur_vy/1 -> cur_vy/1
  Sel_cur_p/1 -> cur_p/1
  Sel_cur_y/1 -> cur_y/1
  vel_in/1 -> Sel_cur_vz/1, Sel_cur_vx/1, Sel_cur_vy/1
  pos_in/1 -> Sel_cur_x/1, Sel_cur_y/1, Sel_cur_z/1
  Sel_cur_x/1 -> cur_x/1
  Sel_cur_q/1 -> cur_q/1
  Sel_cur_r/1 -> cur_r/1
  Sel_cur_vz/1 -> cur_vz/1
  Sel_cur_vx/1 -> cur_vx/1
  Sel_cur_phi/1 -> cur_phi/1
  Sel_cur_theta/1 -> cur_theta/1
  Sel_cur_z/1 -> cur_z/1

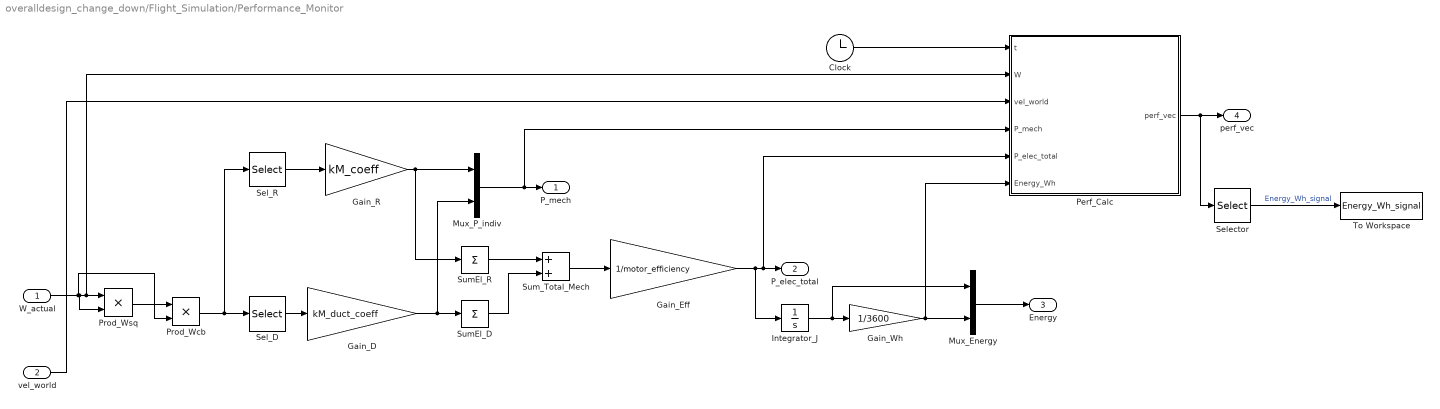
== system overalldesign_change_down/Flight_Simulation/Performance_Monitor ==
  W_actual : Inport
  vel_world : Inport  Port=2  PortDimensions=3
  Clock : Clock
  Gain_D : Gain  Gain=kM_duct_coeff
  Gain_Eff : Gain  Gain=1/motor_efficiency
  Gain_R : Gain  Gain=kM_coeff
  Gain_Wh : Gain  Gain=1/3600
  Integrator_J : Integrator
  Mux_Energy : Mux  Inputs=2
  Mux_P_indiv : Mux  Inputs=2
  Perf_Calc : MATLAB Function  TreatAsAtomicUnit=on
  Prod_Wcb : Product
  Prod_Wsq : Product
  Sel_D : Selector  InputPortWidth=8  IndexOptions=Index vector (dialog)  Indices=[7 8]  OutputSizes=1
  Sel_R : Selector  InputPortWidth=8  IndexOptions=Index vector (dialog)  Indices=[1 2 3 4 5 6]  OutputSizes=1
  Selector : Selector  InputPortWidth=20  IndexOptions=Index vector (dialog)  Indices=13  OutputSizes=1
  SumEl_D : Sum  Inputs=+
  SumEl_R : Sum  Inputs=+
  Sum_Total_Mech : Sum
  To Workspace : ToWorkspace  VariableName=Energy_Wh_signal  SaveFormat=Timeseries  SampleTime=-1
  P_mech : Outport
  P_elec_total : Outport  Port=2
  Energy : Outport  Port=3
  perf_vec : Outport  Port=4
  wires:
  Sel_R/1 -> Gain_R/1
  Prod_Wcb/1 -> Sel_R/1, Sel_D/1
  W_actual/1 -> Perf_Calc/2(W), Prod_Wsq/1, Prod_Wsq/2, Prod_Wcb/2
  Gain_Wh/1 -> Mux_Energy/2, Perf_Calc/6(Energy_Wh)
  Mux_P_indiv/1 -> P_mech/1, Perf_Calc/4(P_mech)
  Gain_Eff/1 -> Perf_Calc/5(P_elec_total), P_elec_total/1, Integrator_J/1
  Prod_Wsq/1 -> Prod_Wcb/1
  Gain_D/1 -> SumEl_D/1, Mux_P_indiv/2
  Gain_R/1 -> SumEl_R/1, Mux_P_indiv/1
  Sel_D/1 -> Gain_D/1
  SumEl_R/1 -> Sum_Total_Mech/1
  SumEl_D/1 -> Sum_Total_Mech/2
  Mux_Energy/1 -> Energy/1
  Sum_Total_Mech/1 -> Gain_Eff/1
  Integrator_J/1 -> Gain_Wh/1, Mux_Energy/1
  Clock/1 -> Perf_Calc/1(t)
  vel_world/1 -> Perf_Calc/3(vel_world)
  Perf_Calc/1(perf_vec) -> Selector/1, perf_vec/1
  Selector/1 -> To Workspace/1  "Energy_Wh_signal"

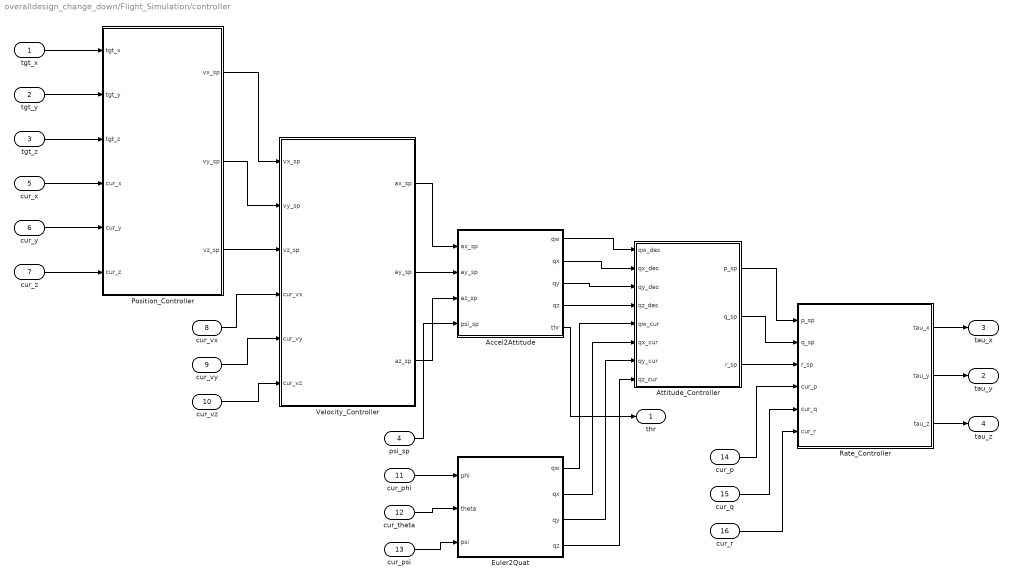
== system overalldesign_change_down/Flight_Simulation/controller ==
  tgt_x : Inport
  tgt_y : Inport  Port=2
  tgt_z : Inport  Port=3
  psi_sp : Inport  Port=4
  cur_x : Inport  Port=5
  cur_y : Inport  Port=6
  cur_z : Inport  Port=7
  cur_vx : Inport  Port=8
  cur_vy : Inport  Port=9
  cur_vz : Inport  Port=10
  cur_phi : Inport  Port=11
  cur_theta : Inport  Port=12
  cur_psi : Inport  Port=13
  cur_p : Inport  Port=14
  cur_q : Inport  Port=15
  cur_r : Inport  Port=16
  Accel2Attitude : Subsystem
  Attitude_Controller : Subsystem
  Euler2Quat : Subsystem
  Position_Controller : Subsystem
  Rate_Controller : Subsystem
  Velocity_Controller : Subsystem
  thr : Outport
  tau_y : Outport  Port=2
  tau_x : Outport  Port=3
  tau_z : Outport  Port=4
  wires:
  tgt_x/1 -> Position_Controller/1(tgt_x)
  cur_theta/1 -> Euler2Quat/2(theta)
  tgt_z/1 -> Position_Controller/3(tgt_z)
  Euler2Quat/2(qx) -> Attitude_Controller/6(qx_cur)
  tgt_y/1 -> Position_Controller/2(tgt_y)
  cur_p/1 -> Rate_Controller/4(cur_p)
  cur_z/1 -> Position_Controller/6(cur_z)
  cur_x/1 -> Position_Controller/4(cur_x)
  cur_y/1 -> Position_Controller/5(cur_y)
  Position_Controller/2(vy_sp) -> Velocity_Controller/2(vy_sp)
  Attitude_Controller/3(r_sp) -> Rate_Controller/3(r_sp)
  Position_Controller/1(vx_sp) -> Velocity_Controller/1(vx_sp)
  Position_Controller/3(vz_sp) -> Velocity_Controller/3(vz_sp)
  cur_vx/1 -> Velocity_Controller/4(cur_vx)
  cur_vy/1 -> Velocity_Controller/5(cur_vy)
  Attitude_Controller/2(q_sp) -> Rate_Controller/2(q_sp)
  cur_vz/1 -> Velocity_Controller/6(cur_vz)
  Velocity_Controller/1(ax_sp) -> Accel2Attitude/1(ax_sp)
  Rate_Controller/3(tau_z) -> tau_z/1
  Rate_Controller/2(tau_y) -> tau_y/1
  Velocity_Controller/2(ay_sp) -> Accel2Attitude/2(ay_sp)
  Velocity_Controller/3(az_sp) -> Accel2Attitude/3(az_sp)
  cur_q/1 -> Rate_Controller/5(cur_q)
  psi_sp/1 -> Accel2Attitude/4(psi_sp)
  cur_phi/1 -> Euler2Quat/1(phi)
  cur_psi/1 -> Euler2Quat/3(psi)
  Accel2Attitude/1(qw) -> Attitude_Controller/1(qw_des)
  Accel2Attitude/2(qx) -> Attitude_Controller/2(qx_des)
  Accel2Attitude/3(qy) -> Attitude_Controller/3(qy_des)
  Accel2Attitude/4(qz) -> Attitude_Controller/4(qz_des)
  Accel2Attitude/5(thr) -> thr/1
  Euler2Quat/1(qw) -> Attitude_Controller/5(qw_cur)
  Euler2Quat/3(qy) -> Attitude_Controller/7(qy_cur)
  Euler2Quat/4(qz) -> Attitude_Controller/8(qz_cur)
  Attitude_Controller/1(p_sp) -> Rate_Controller/1(p_sp)
  cur_r/1 -> Rate_Controller/6(cur_r)
  Rate_Controller/1(tau_x) -> tau_x/1

== system overalldesign_change_down/Flight_Simulation/mixer ==
  T_des : Inport
  tau_y : Inport  Port=2
  tau_x : Inport  Port=3
  tau_z : Inport  Port=4
  CGoffset : Inport  Port=5
  motor_coord : Inport  Port=6
  fault_id : Constant  Value=0  VectorParams1D=off
  mixer_fcn : MATLAB Function  TreatAsAtomicUnit=on
  W : Outport  PortDimensions=8
  wires:
  CGoffset/1 -> mixer_fcn/6(CGoffset)
  tau_z/1 -> mixer_fcn/4(tau_z)
  tau_x/1 -> mixer_fcn/3(tau_x)
  tau_y/1 -> mixer_fcn/2(tau_y)
  T_des/1 -> mixer_fcn/1(T_des)
  mixer_fcn/1(W) -> W/1
  fault_id/1 -> mixer_fcn/5(fault_id)
  motor_coord/1 -> mixer_fcn/7(motor_coord)

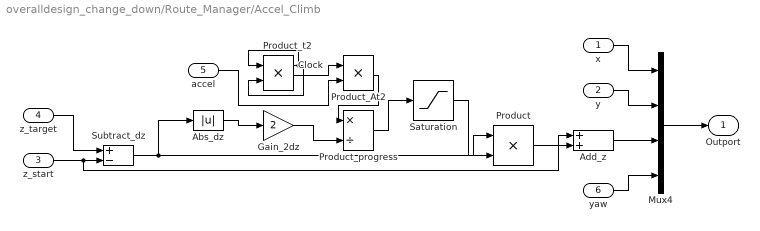
== system overalldesign_change_down/Route_Manager/Accel_Climb ==
  x : Inport
  y : Inport  Port=2
  z_start : Inport  Port=3
  z_target : Inport  Port=4
  accel : Inport  Port=5
  yaw : Inport  Port=6
  Abs_dz : Abs  SaturateOnIntegerOverflow=off
  Add_z : Sum
  Clock : Clock
  Gain_2dz : Gain  Gain=2
  Mux4 : Mux
  Product : Product  Inputs=**
  Product_At2 : Product  Inputs=**
  Product_progress : Product  Inputs=*/
  Product_t2 : Product  Inputs=**
  Saturation : Saturate  UpperLimit=1  LowerLimit=0
  Subtract_dz : Sum  Inputs=+-
  Outport : Outport
  wires:
  Clock/1 -> Product_t2/1, Product_t2/2
  Product_t2/1 -> Product_At2/1
  accel/1 -> Product_At2/2
  z_start/1 -> Add_z/1, Subtract_dz/2
  Subtract_dz/1 -> Abs_dz/1, Product/1
  Abs_dz/1 -> Gain_2dz/1
  Product_At2/1 -> Product_progress/1
  Gain_2dz/1 -> Product_progress/2
  Product_progress/1 -> Saturation/1
  Saturation/1 -> Product/2
  Product/1 -> Add_z/2
  x/1 -> Mux4/1
  y/1 -> Mux4/2
  Add_z/1 -> Mux4/3
  yaw/1 -> Mux4/4
  Mux4/1 -> Outport/1
  z_target/1 -> Subtract_dz/1

== system overalldesign_change_down/Route_Manager/Accel_Descend ==
  x : Inport
  y : Inport  Port=2
  z0 : Inport  Port=3
  V_descent : Inport  Port=4
  a_brake : Inport  Port=5
  yaw : Inport  Port=6
  Clock : Clock
  Mux4 : Mux
  descend_profile : MATLAB Function  TreatAsAtomicUnit=on
  Outport : Outport
  wires:
  y/1 -> Mux4/2
  Clock/1 -> descend_profile/1(t_clock)
  z0/1 -> descend_profile/2(z0)
  x/1 -> Mux4/1
  a_brake/1 -> descend_profile/4(a_brake)
  descend_profile/1(z) -> Mux4/3
  yaw/1 -> Mux4/4
  Mux4/1 -> Outport/1
  V_descent/1 -> descend_profile/3(V_descent)

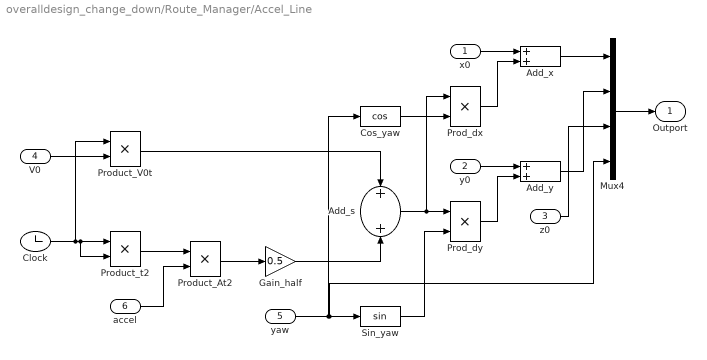
== system overalldesign_change_down/Route_Manager/Accel_Line ==
  x0 : Inport
  y0 : Inport  Port=2
  z0 : Inport  Port=3
  V0 : Inport  Port=4
  yaw : Inport  Port=5
  accel : Inport  Port=6
  Add_s : Sum
  Add_x : Sum
  Add_y : Sum
  Clock : Clock
  Cos_yaw : Trigonometry  Operator=cos
  Gain_half : Gain  Gain=0.5
  Mux4 : Mux
  Prod_dx : Product  Inputs=**
  Prod_dy : Product  Inputs=**
  Product_At2 : Product  Inputs=**
  Product_V0t : Product  Inputs=**
  Product_t2 : Product  Inputs=**
  Sin_yaw : Trigonometry
  Outport : Outport
  wires:
  Clock/1 -> Product_t2/2, Product_t2/1, Product_V0t/1
  yaw/1 -> Mux4/4, Sin_yaw/1, Cos_yaw/1
  Add_s/1 -> Prod_dx/1, Prod_dy/1
  Gain_half/1 -> Add_s/2
  accel/1 -> Product_At2/2
  Add_y/1 -> Mux4/2
  V0/1 -> Product_V0t/2
  Product_At2/1 -> Gain_half/1
  Prod_dx/1 -> Add_x/2
  Product_t2/1 -> Product_At2/1
  Mux4/1 -> Outport/1
  Product_V0t/1 -> Add_s/1
  Cos_yaw/1 -> Prod_dx/2
  Sin_yaw/1 -> Prod_dy/2
  x0/1 -> Add_x/1
  Add_x/1 -> Mux4/1
  y0/1 -> Add_y/1
  Prod_dy/1 -> Add_y/2
  z0/1 -> Mux4/3

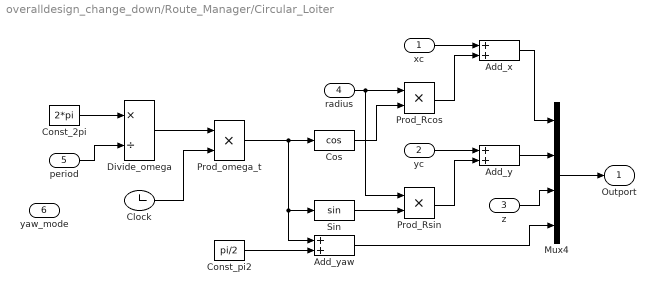
== system overalldesign_change_down/Route_Manager/Circular_Loiter ==
  xc : Inport
  yc : Inport  Port=2
  z : Inport  Port=3
  radius : Inport  Port=4
  period : Inport  Port=5
  yaw_mode : Inport  Port=6
  Add_x : Sum
  Add_y : Sum
  Add_yaw : Sum
  Clock : Clock
  Const_2pi : Constant  Value=2*pi
  Const_pi2 : Constant  Value=pi/2
  Cos : Trigonometry  Operator=cos
  Divide_omega : Product  Inputs=*/
  Mux4 : Mux
  Prod_Rcos : Product  Inputs=**
  Prod_Rsin : Product  Inputs=**
  Prod_omega_t : Product  Inputs=**
  Sin : Trigonometry
  Outport : Outport
  wires:
  Clock/1 -> Prod_omega_t/2
  Sin/1 -> Prod_Rsin/2
  Divide_omega/1 -> Prod_omega_t/1
  Const_2pi/1 -> Divide_omega/1
  period/1 -> Divide_omega/2
  Const_pi2/1 -> Add_yaw/2
  Prod_omega_t/1 -> Sin/1, Add_yaw/1, Cos/1
  radius/1 -> Prod_Rsin/1, Prod_Rcos/1
  Cos/1 -> Prod_Rcos/2
  Add_yaw/1 -> Mux4/4
  xc/1 -> Add_x/1
  Mux4/1 -> Outport/1
  Prod_Rcos/1 -> Add_x/2
  yc/1 -> Add_y/1
  Prod_Rsin/1 -> Add_y/2
  Add_x/1 -> Mux4/1
  Add_y/1 -> Mux4/2
  z/1 -> Mux4/3

== system overalldesign_change_down/Route_Manager/Hover ==
  x : Inport
  y : Inport  Port=2
  z : Inport  Port=3
  yaw : Inport  Port=4
  Mux4 : Mux
  Outport : Outport
  wires:
  x/1 -> Mux4/1
  y/1 -> Mux4/2
  z/1 -> Mux4/3
  yaw/1 -> Mux4/4
  Mux4/1 -> Outport/1

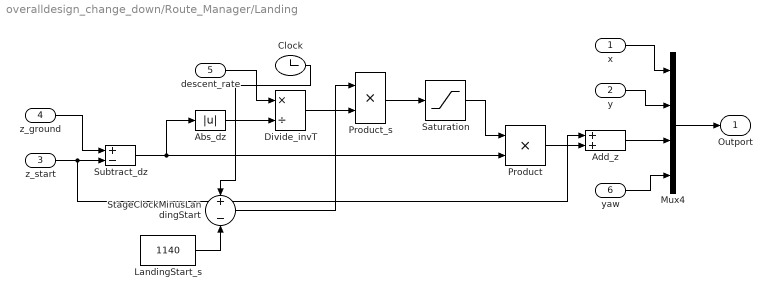
== system overalldesign_change_down/Route_Manager/Landing ==
  x : Inport
  y : Inport  Port=2
  z_start : Inport  Port=3
  z_ground : Inport  Port=4
  descent_rate : Inport  Port=5
  yaw : Inport  Port=6
  Abs_dz : Abs  SaturateOnIntegerOverflow=off
  Add_z : Sum
  Clock : Clock
  Divide_invT : Product  Inputs=*/
  LandingStart_s : Constant  Value=1140
  Mux4 : Mux
  Product : Product  Inputs=**
  Product_s : Product  Inputs=**
  Saturation : Saturate  UpperLimit=1  LowerLimit=0
  StageClockMinusLandingStart : Sum  Inputs=+-
  Subtract_dz : Sum  Inputs=+-
  Outport : Outport
  wires:
  z_ground/1 -> Subtract_dz/1
  Product_s/1 -> Saturation/1
  Divide_invT/1 -> Product_s/2
  Abs_dz/1 -> Divide_invT/2
  z_start/1 -> Subtract_dz/2, Add_z/1
  Subtract_dz/1 -> Product/2, Abs_dz/1
  descent_rate/1 -> Divide_invT/1
  Add_z/1 -> Mux4/3
  Saturation/1 -> Product/1
  Product/1 -> Add_z/2
  x/1 -> Mux4/1
  y/1 -> Mux4/2
  yaw/1 -> Mux4/4
  Mux4/1 -> Outport/1
  Clock/1 -> StageClockMinusLandingStart/1
  LandingStart_s/1 -> StageClockMinusLandingStart/2
  StageClockMinusLandingStart/1 -> Product_s/1

== system overalldesign_change_down/Route_Manager/Line_Cruise ==
  x0 : Inport
  y0 : Inport  Port=2
  z0 : Inport  Port=3
  speed : Inport  Port=4
  yaw : Inport  Port=5
  Clock : Clock
  Mux4 : Mux
  smooth_cruise : MATLAB Function  TreatAsAtomicUnit=on
  Outport : Outport
  wires:
  Clock/1 -> smooth_cruise/1(t_clock)
  x0/1 -> smooth_cruise/2(x0)
  y0/1 -> smooth_cruise/3(y0)
  speed/1 -> smooth_cruise/4(speed)
  yaw/1 -> smooth_cruise/5(yaw), Mux4/4
  smooth_cruise/1(x) -> Mux4/1
  smooth_cruise/2(y) -> Mux4/2
  z0/1 -> Mux4/3
  Mux4/1 -> Outport/1

== system overalldesign_change_down/Route_Manager/Takeoff ==
  x : Inport
  y : Inport  Port=2
  z_start : Inport  Port=3
  z_target : Inport  Port=4
  climb_rate : Inport  Port=5
  yaw : Inport  Port=6
  Clock : Clock
  Mux4 : Mux
  smooth_takeoff : MATLAB Function  TreatAsAtomicUnit=on
  Outport : Outport
  wires:
  x/1 -> Mux4/1
  y/1 -> Mux4/2
  smooth_takeoff/1(z) -> Mux4/3
  yaw/1 -> Mux4/4
  Mux4/1 -> Outport/1
  Clock/1 -> smooth_takeoff/1(t_clock)
  z_start/1 -> smooth_takeoff/2(z_start)
  z_target/1 -> smooth_takeoff/3(z_target)
  climb_rate/1 -> smooth_takeoff/4(climb_rate)

== system overalldesign_change_down/Flight_Simulation/Dynamics_Subsys/Aero_Model ==
  V_body : Inport
  euler : Inport  Port=2
  MATLAB Function : MATLAB Function  TreatAsAtomicUnit=on
  F_aero : Outport
  M_aero : Outport  Port=2
  wires:
  V_body/1 -> MATLAB Function/1(V_body)
  euler/1 -> MATLAB Function/2(euler)
  MATLAB Function/1(F_aero) -> F_aero/1
  MATLAB Function/2(M_aero) -> M_aero/1

== system overalldesign_change_down/Flight_Simulation/controller/Accel2Attitude ==
  ax_sp : Inport
  ay_sp : Inport  Port=2
  az_sp : Inport  Port=3
  psi_sp : Inport  Port=4
  accel2quat : MATLAB Function  TreatAsAtomicUnit=on
  qw : Outport
  qx : Outport  Port=2
  qy : Outport  Port=3
  qz : Outport  Port=4
  thr : Outport  Port=5
  wires:
  ax_sp/1 -> accel2quat/1(ax)
  ay_sp/1 -> accel2quat/2(ay)
  accel2quat/3(qy) -> qy/1
  az_sp/1 -> accel2quat/3(az)
  accel2quat/4(qz) -> qz/1
  accel2quat/1(qw) -> qw/1
  psi_sp/1 -> accel2quat/4(psi)
  accel2quat/2(qx) -> qx/1
  accel2quat/5(thr) -> thr/1

== system overalldesign_change_down/Flight_Simulation/controller/Attitude_Controller ==
  qw_des : Inport
  qx_des : Inport  Port=2
  qy_des : Inport  Port=3
  qz_des : Inport  Port=4
  qw_cur : Inport  Port=5
  qx_cur : Inport  Port=6
  qy_cur : Inport  Port=7
  qz_cur : Inport  Port=8
  quat_att_control : MATLAB Function  TreatAsAtomicUnit=on
  p_sp : Outport
  q_sp : Outport  Port=2
  r_sp : Outport  Port=3
  wires:
  qx_cur/1 -> quat_att_control/6(qx_cur)
  qw_des/1 -> quat_att_control/1(qw_des)
  qw_cur/1 -> quat_att_control/5(qw_cur)
  qx_des/1 -> quat_att_control/2(qx_des)
  qz_cur/1 -> quat_att_control/8(qz_cur)
  qy_des/1 -> quat_att_control/3(qy_des)
  qz_des/1 -> quat_att_control/4(qz_des)
  qy_cur/1 -> quat_att_control/7(qy_cur)
  quat_att_control/1(p_sp) -> p_sp/1
  quat_att_control/2(q_sp) -> q_sp/1
  quat_att_control/3(r_sp) -> r_sp/1

== system overalldesign_change_down/Flight_Simulation/controller/Euler2Quat ==
  phi : Inport
  theta : Inport  Port=2
  psi : Inport  Port=3
  euler2quat : MATLAB Function  TreatAsAtomicUnit=on
  qw : Outport
  qx : Outport  Port=2
  qy : Outport  Port=3
  qz : Outport  Port=4
  wires:
  euler2quat/2(qx) -> qx/1
  phi/1 -> euler2quat/1(phi)
  euler2quat/1(qw) -> qw/1
  psi/1 -> euler2quat/3(psi)
  theta/1 -> euler2quat/2(theta)
  euler2quat/3(qy) -> qy/1
  euler2quat/4(qz) -> qz/1

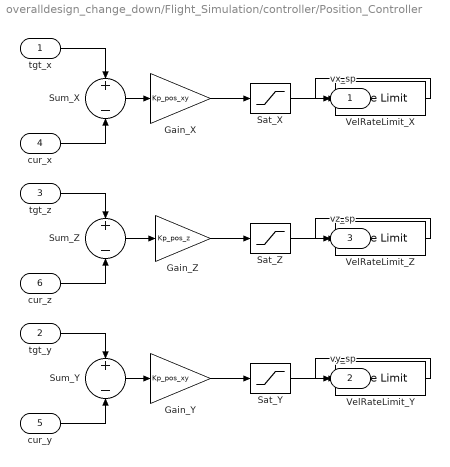
== system overalldesign_change_down/Flight_Simulation/controller/Position_Controller ==
  tgt_x : Inport
  tgt_y : Inport  Port=2
  tgt_z : Inport  Port=3
  cur_x : Inport  Port=4
  cur_y : Inport  Port=5
  cur_z : Inport  Port=6
  Gain_X : Gain  Gain=Kp_pos_xy
  Gain_Y : Gain  Gain=Kp_pos_xy
  Gain_Z : Gain  Gain=Kp_pos_z
  Sat_X : Saturate  UpperLimit=CS_max_vel_xy  LowerLimit=-CS_max_vel_xy
  Sat_Y : Saturate  UpperLimit=CS_max_vel_xy  LowerLimit=-CS_max_vel_xy
  Sat_Z : Saturate  UpperLimit=CS_max_vel_z_up  LowerLimit=-CS_max_vel_z_down
  Sum_X : Sum  Inputs=+-
  Sum_Y : Sum  Inputs=+-
  Sum_Z : Sum  Inputs=+-
  VelRateLimit_X : RateLimiter  RisingSlewLimit=CS_max_acc_xy  FallingSlewLimit=-CS_max_acc_xy  SampleTimeMode=inherited
  VelRateLimit_Y : RateLimiter  RisingSlewLimit=CS_max_acc_xy  FallingSlewLimit=-CS_max_acc_xy  SampleTimeMode=inherited
  VelRateLimit_Z : RateLimiter  RisingSlewLimit=CS_max_acc_z_up  FallingSlewLimit=-CS_max_acc_z_down  SampleTimeMode=inherited
  vx_sp : Outport
  vy_sp : Outport  Port=2
  vz_sp : Outport  Port=3
  wires:
  cur_y/1 -> Sum_Y/2
  tgt_y/1 -> Sum_Y/1
  cur_z/1 -> Sum_Z/2
  tgt_z/1 -> Sum_Z/1
  cur_x/1 -> Sum_X/2
  Gain_Y/1 -> Sat_Y/1
  tgt_x/1 -> Sum_X/1
  Sum_Z/1 -> Gain_Z/1
  Sum_X/1 -> Gain_X/1
  Sum_Y/1 -> Gain_Y/1
  Gain_X/1 -> Sat_X/1
  Gain_Z/1 -> Sat_Z/1
  Sat_X/1 -> VelRateLimit_X/1
  VelRateLimit_X/1 -> vx_sp/1
  Sat_Y/1 -> VelRateLimit_Y/1
  VelRateLimit_Y/1 -> vy_sp/1
  Sat_Z/1 -> VelRateLimit_Z/1
  VelRateLimit_Z/1 -> vz_sp/1
